simulink model "PDGF"  (R2021b)
settings: Solver=VariableStepAuto  StartTime=0.0  StopTime=15  RelTol=1e-3
values from neighbouring files (symbols this model uses):
  dq_i = [0,0,0]    [param.m]
  F_v = zeros(3,3)    [param.m]
  K_d = diag([50 50 50])    [param.m]
  K_p = diag([200 200 200])    [param.m]
  q_f = [0.1,0.1,0.1]    [param.m]
  q_i = [0,0,0,]    [param.m]
settings Model: Creator=ASUS  LastModifiedBy=ASUS

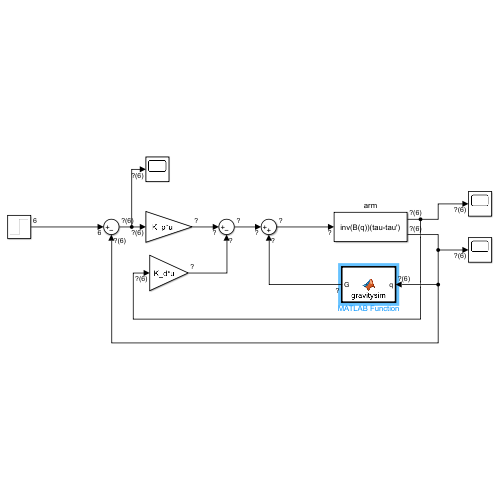
[thumbnail: Simulink's stored preview of the top-level diagram]
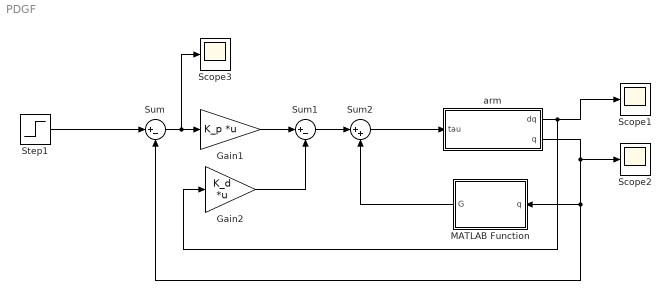
== system PDGF ==
  Gain1 : Gain  Gain=K_p  Multiplication=Matrix(K*u)
  Gain2 : Gain  Gain=K_d  Multiplication=Matrix(K*u)
  MATLAB Function : MATLAB Function  TreatAsAtomicUnit=on
  Scope1 : Scope
  Scope2 : Scope
  Scope3 : Scope
  Step1 : Step  Time=0  Before=q_i  After=q_f  SampleTime=0
  Sum : Sum  Inputs=|+-
  Sum1 : Sum  Inputs=|+-
  Sum2 : Sum  Inputs=|++
  arm : Subsystem
      mask Display: disp('inv(B(q))(tau-tau'')')
  wires:
  Sum1/1 -> Sum2/1
  Sum2/1 -> arm/1(tau)
  arm/1(dq) -> Gain2/1, Scope1/1
  Sum/1 -> Scope3/1, Gain1/1
  Step1/1 -> Sum/1
  arm/2("q ") -> Sum/2, MATLAB Function/1(q), Scope2/1
  MATLAB Function/1(G) -> Sum2/2
  Gain1/1 -> Sum1/1
  Gain2/1 -> Sum1/2

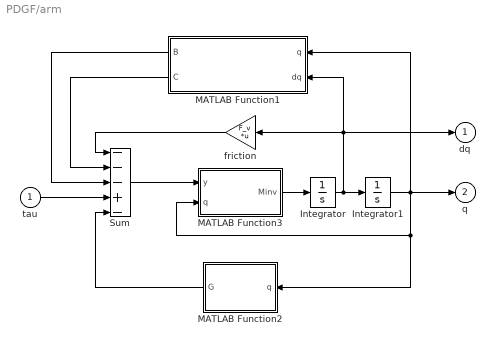
== system PDGF/arm ==
  tau : Inport
  Integrator : Integrator  InitialCondition=dq_i  ZeroCross=off
  Integrator1 : Integrator  InitialCondition=q_i  ZeroCross=off
  MATLAB Function1 : MATLAB Function  TreatAsAtomicUnit=on
  MATLAB Function2 : MATLAB Function  TreatAsAtomicUnit=on
  MATLAB Function3 : MATLAB Function  TreatAsAtomicUnit=on
  Sum : Sum  Inputs=---+-  InputSameDT=on  SaturateOnIntegerOverflow=on  OutDataTypeStr=Inherit: Same as first input
  friction : Gain  Gain=F_v  Multiplication=Matrix(K*u)  SaturateOnIntegerOverflow=on  OutDataTypeStr=Inherit: Same as input  ParamDataTypeStr=Inherit: Same as input
      mask Display: disp('F_v')
  dq : Outport  InitialOutput=0
  "q " : Outport  Port=2  InitialOutput=0
  wires:
  Integrator1/1 -> MATLAB Function1/1(q), MATLAB Function2/1(q), MATLAB Function3/2(q), "q "/1
  MATLAB Function3/1(Minv) -> Integrator/1
  Integrator/1 -> Integrator1/1, dq/1, MATLAB Function1/2(dq), friction/1
  Sum/1 -> MATLAB Function3/1(y)
  friction/1 -> Sum/1
  MATLAB Function2/1(G) -> Sum/5
  tau/1 -> Sum/4
  MATLAB Function1/1(B) -> Sum/3
  MATLAB Function1/2(C) -> Sum/2

== matlab function PDGF/arm/MATLAB Function1 ==
  data: q input; B output; dq input; C output
function [B,C] = corioliscentrifugalsim(q, dq)
[B,C] = corioliscentrifugal(q, dq);
end

== matlab function PDGF/arm/MATLAB Function2 ==
  data: q input; G output
function G = gravitysim(q)
G = gravity(q);
end

== matlab function PDGF/arm/MATLAB Function3 ==
  data: y input; q input; Minv output
function Minv = inertiainvsim(y, q)
M = inertia(q);
% M=M(1:3,1:3);
Minv = inv(M)*y;

end

== matlab function PDGF/MATLAB Function ==
  data: q input; G output
function G = gravitysim(q)
G = gravity(q);
end
